simulink model "Loops9"  (Simulink 8.7)
settings: Solver=ode45  StartTime=0.0  StopTime=10.0  RelTol=1e-3
settings Model: Creator=scaife  LastModifiedBy=bourbouh  ExtModeAutoUpdateStatusClock=off
settings DataIOCC: SignalLoggingSaveFormat=ModelDataLogs  SignalLoggingName=sigsOut
settings OptimizationCC: InitFltsAndDblsToZero=on
settings DebuggingCC: SaveWithParameterizedLinksMsg=none  SignalResolutionControl=TryResolveAllWithWarning  MultiTaskDSMMsg=warning  MultiTaskCondExecSysMsg=none
settings HardwareCC: TargetUnknown=on
settings SFSimCC: SimParseCustomCode=off
settings GRTTargetCC: TargetFcnLib=ansi_tfl_tmw.mat  ModelReferenceCompliant=off  GeneratePreprocessorConditionals=Use local settings  CombineOutputUpdateFcns=off  MatFileLogging=off  GRTInterface=on

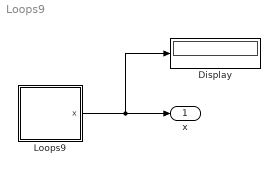
== system Loops9 ==
  Display : Display
  Loops9 : Stateflow chart  TreatAsAtomicUnit=on
  x : Outport
  wires:
  Loops9/1(x) -> Display/1, x/1

== stateflow chart Loops9 ==
  state A
  state B
  (default) -> A
  (junction 6) -> A [order 2]
  A -> (junction 6) : {x=0}
  (junction 7) -> (junction 6) [order 2]
  (junction 6) -> (junction 7) [order 1] : [x==0]
  (junction 7) -> B [order 1] : [x==0]
  B -> (junction 7) : {x=1}
  data: x output int32
